simulink model "strejc"  (R2012a)
settings: Solver=ode45  SolverMode=SingleTasking  StartTime=0.0  StopTime=t_sym  RelTol=1e-3
settings Model: CovMetricSettings=dwe  CovHtmlReporting=off  covSaveCumulativeToWorkspaceVar=off  CovSaveSingleToWorkspaceVar=off  CovExternalEMLEnable=on  Creator=rafal  LastModifiedBy=rafal
settings DataIOCC: SaveFormat=StructureWithTime  ReturnWorkspaceOutputs=off
settings OptimizationCC: LifeSpan=inf  SimCompilerOptimization=Off
settings DebuggingCC: FcnCallInpInsideContextMsg=Enable All
settings HardwareCC: ProdWordSize=32  ProdHWDeviceType=Specified
settings SFSimCC: SimUseLocalCustomCode=off
settings RTWCC: RTWUseLocalCustomCode=off  RTWCompilerOptimization=Off
settings GRTTargetCC: CodeReplacementLibrary=C99 (ISO)  CPPClassGenCompliant=off

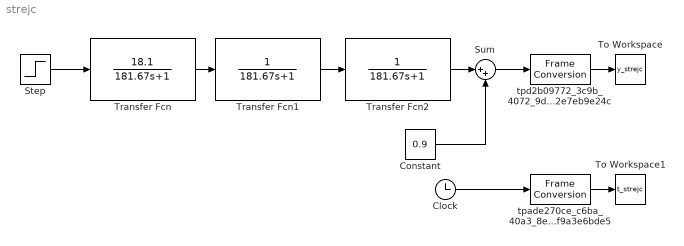
== system strejc ==
  Clock : Clock
  Constant : Constant  Value=0.9
  "Step " : Step  Time=29.025  SampleTime=0
  Sum : Sum  Inputs=|++
  To Workspace : ToWorkspace  VariableName=y_strejc  SampleTime=-1
  To Workspace1 : ToWorkspace  VariableName=t_strejc  SampleTime=-1
  Transfer Fcn : TransferFcn  Numerator=[18.1]  Denominator=[181.67 1]
  Transfer Fcn1 : TransferFcn  Denominator=[181.67 1]
  Transfer Fcn2 : TransferFcn  Denominator=[181.67 1]
  tpade270ce_c6ba_40a3_8e1c_34f9a3e6bde5 : FrameConversion  OutFrame=Sample-based
  tpd2b09772_3c9b_4072_9def_9e2e7eb9e24c : FrameConversion  OutFrame=Sample-based
  wires:
  "Step "/1 -> Transfer Fcn/1
  Transfer Fcn/1 -> Transfer Fcn1/1
  Transfer Fcn1/1 -> Transfer Fcn2/1
  Transfer Fcn2/1 -> Sum/1
  Constant/1 -> Sum/2
  Sum/1 -> tpd2b09772_3c9b_4072_9def_9e2e7eb9e24c/1
  tpd2b09772_3c9b_4072_9def_9e2e7eb9e24c/1 -> To Workspace/1
  Clock/1 -> tpade270ce_c6ba_40a3_8e1c_34f9a3e6bde5/1
  tpade270ce_c6ba_40a3_8e1c_34f9a3e6bde5/1 -> To Workspace1/1
